simulink library "Common_Library"  (Simulink 8.1)
settings: Solver=ode45  StartTime=0.0  StopTime=10.0  RelTol=1e-3
values from neighbouring files (symbols this model uses):
  address_0x00 = MOVcr    [ROM.m]
  address_0x01 = 10    [ROM.m]
  address_0x02 = REG_A    [ROM.m]
  address_0x03 = MOVcr    [ROM.m]
  address_0x04 = 3    [ROM.m]
  address_0x05 = REG_B    [ROM.m]
  address_0x06 = ADDcr    [ROM.m]
  address_0x07 = 50    [ROM.m]
  address_0x08 = REG_B    [ROM.m]
  address_0x09 = ADDrr    [ROM.m]
  address_0x0A = REG_A    [ROM.m]
  address_0x0B = REG_B    [ROM.m]
  address_0x0C = 0    [ROM.m]
  address_0x0D = 0    [ROM.m]
  address_0x0E = 0    [ROM.m]
  address_0x0F = 177    [ROM.m]
libraries: Common_Library x115, Computer_Library x85, commutil2 x67, simulink_extras x1
(part 1 of 3)
settings Model: Creator=uzivatel  LastModifiedBy=uzivatel

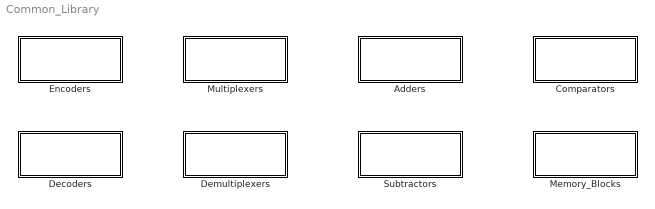
== system Common_Library ==
  Adders : Subsystem
  Comparators : Subsystem
  Decoders : Subsystem
  Demultiplexers : Subsystem
  Encoders : Subsystem
  Memory_Blocks : Subsystem
  Multiplexers : Subsystem
  Subtractors : Subsystem

== system Common_Library/Adders ==
  1_Bit_Adder : Subsystem
  1_Byte_Adder : Subsystem

== system Common_Library/Comparators ==
  1_Bit_Comparator : Subsystem
  1_Byte_Comparator : Subsystem

== system Common_Library/Decoders ==
  2_to_4_Decoder : Subsystem  TreatAsAtomicUnit=on
  3_to_8_Decoder : Subsystem  TreatAsAtomicUnit=on
  4_to_16_Decoder : Subsystem  RequirementInfo={} %GIDa_0eac4206_ee83_4851_a053_5bf277ce373a  TreatAsAtomicUnit=on
  __8_to_256_Decoder__ : Subsystem  Commented=on

== system Common_Library/Demultiplexers ==
  1_to_2_Bit_Demultiplexer : Subsystem
  1_to_2_Byte_Demultiplexer : Subsystem
  1_to_4_Bit_Demultiplexer : Subsystem
  1_to_4_Byte_Demultiplexer : Subsystem
  1_to_8_Bit_Demultiplexer : Subsystem
  1_to_8_Byte_Demultiplexer : Subsystem
  __1_to_16_Bit_Demultiplexer__ : Subsystem  Commented=on
  __1_to_16_Byte_Demultiplexer__ : Subsystem  Commented=on
  __1_to_256_Bit_Demultiplexer__ : Subsystem  Commented=on
  __1_to_256_Byte_Demultiplexer__ : Subsystem  Commented=on

== system Common_Library/Encoders ==
  4_to_2_Encoder : Subsystem
  __16_to_4_Encoder__ : Subsystem  Commented=on
  __8_to_3_Encoder__ : Subsystem  Commented=on

== system Common_Library/Memory_Blocks ==
  16B_RAM_Memory : Subsystem
  16B_ROM_Memory : Subsystem
  Bit : Subsystem
  Byte : Subsystem

== system Common_Library/Multiplexers ==
  16_to_1_Bit_Multiplexer : Subsystem
  16_to_1_Byte_Multiplexer : Subsystem
  2_to_1_Bit_Multiplexer : Subsystem
  2_to_1_Byte_Multiplexer : Subsystem
  4_to_1_Bit_Multiplexer : Subsystem
  4_to_1_Byte_Multiplexer : Subsystem
  8_to_1_Bit_Multiplexer : Subsystem
  8_to_1_Byte_Multiplexer : Subsystem
  __256_to_1_Bit_Multiplexer__ : Subsystem  Commented=on
  __256_to_1_Byte_Multiplexer__ : Subsystem  Commented=on

== system Common_Library/Subtractors ==
  1_Bit_Subtractor : Subsystem
  1_Byte_Subtractor : Subsystem

== system Common_Library/Adders/1_Bit_Adder ==
  Data_In_A(1b) : Inport
  Data_In_B(1b) : Inport  Port=2
  Carry_In(1b) : Inport  Port=3
  Logical Operator : Logic  IconShape=distinctive  AllPortsSameDT=off  OutDataTypeStr=boolean
  Logical Operator1 : Logic  IconShape=distinctive  AllPortsSameDT=off  OutDataTypeStr=boolean
  Logical Operator10 : Logic  Operator=NOT  Inputs=4  IconShape=distinctive  AllPortsSameDT=off  OutDataTypeStr=boolean
  Logical Operator11 : Logic  Operator=NOT  Inputs=4  IconShape=distinctive  AllPortsSameDT=off  OutDataTypeStr=boolean
  Logical Operator2 : Logic  IconShape=distinctive  AllPortsSameDT=off  OutDataTypeStr=boolean
  Logical Operator{3..6} (4 alike) : Logic  Inputs=3  IconShape=distinctive  AllPortsSameDT=off  OutDataTypeStr=boolean
  Logical Operator7 : Logic  Operator=OR  Inputs=4  IconShape=distinctive  AllPortsSameDT=off  OutDataTypeStr=boolean
  Logical Operator8 : Logic  Operator=OR  Inputs=3  IconShape=distinctive  AllPortsSameDT=off  OutDataTypeStr=boolean
  Logical Operator9 : Logic  Operator=NOT  Inputs=4  IconShape=distinctive  AllPortsSameDT=off  OutDataTypeStr=boolean
  Data_Out(1b) : Outport
  Carry_Out(1b) : Outport  Port=2
  wires:
  Logical Operator11/1 -> Logical Operator4/3, Logical Operator5/3
  Logical Operator10/1 -> Logical Operator3/2, Logical Operator5/2
  Logical Operator9/1 -> Logical Operator3/1, Logical Operator4/1
  Data_In_A(1b)/1 -> Logical Operator9/1, Logical Operator5/1, Logical Operator6/1, Logical Operator/1, Logical Operator1/1
  Data_In_B(1b)/1 -> Logical Operator10/1, Logical Operator4/2, Logical Operator6/2, Logical Operator/2, Logical Operator2/1
  Carry_In(1b)/1 -> Logical Operator11/1, Logical Operator3/3, Logical Operator6/3, Logical Operator1/2, Logical Operator2/2
  Logical Operator2/1 -> Logical Operator8/3
  Logical Operator1/1 -> Logical Operator8/2
  Logical Operator/1 -> Logical Operator8/1
  Logical Operator8/1 -> Carry_Out(1b)/1
  Logical Operator7/1 -> Data_Out(1b)/1
  Logical Operator6/1 -> Logical Operator7/4
  Logical Operator5/1 -> Logical Operator7/3
  Logical Operator4/1 -> Logical Operator7/2
  Logical Operator3/1 -> Logical Operator7/1

== system Common_Library/Adders/1_Byte_Adder ==
  Data_In_A(1B) : Inport
  Data_In_B(1B) : Inport  Port=2
  1_Bit_Adder{0..7} (8 alike) : Common_Library/Adders/1_Bit_Adder
  Bit to Integer Converter : commutil2/Bit to Integer Converter  nbits=8  bitOrder=MSB first  signedOutputValues=Unsigned  outDtype=uint8  outDtypeSigned=Inherit via internal rule
  Constant : Constant  Value=0
  Demux : Demux  Outputs=8
  Demux1 : Demux  Outputs=8
  Integer to Bit Converter : commutil2/Integer to Bit Converter  nbits=8  signedInputValues=Unsigned  bitOrder=MSB first  outDtype=uint8
  Integer to Bit Converter1 : commutil2/Integer to Bit Converter  nbits=8  signedInputValues=Unsigned  bitOrder=MSB first  outDtype=uint8
  Mux : Mux  Inputs=8
  Data_Out(1B) : Outport
  Carry_Out(1b) : Outport  Port=2
  wires:
  Bit to Integer Converter/1 -> Data_Out(1B)/1
  Mux/1 -> Bit to Integer Converter/1
  Integer to Bit Converter1/1 -> Demux1/1
  Data_In_B(1B)/1 -> Integer to Bit Converter1/1
  Integer to Bit Converter/1 -> Demux/1
  Data_In_A(1B)/1 -> Integer to Bit Converter/1
  1_Bit_Adder6/2 -> 1_Bit_Adder7/3
  1_Bit_Adder5/2 -> 1_Bit_Adder6/3
  1_Bit_Adder4/2 -> 1_Bit_Adder5/3
  1_Bit_Adder3/2 -> 1_Bit_Adder4/3
  1_Bit_Adder2/2 -> 1_Bit_Adder3/3
  1_Bit_Adder1/2 -> 1_Bit_Adder2/3
  1_Bit_Adder0/2 -> 1_Bit_Adder1/3
  1_Bit_Adder7/2 -> Carry_Out(1b)/1
  Constant/1 -> 1_Bit_Adder0/3
  Demux1/8 -> 1_Bit_Adder0/2
  Demux1/7 -> 1_Bit_Adder1/2
  Demux1/6 -> 1_Bit_Adder2/2
  Demux1/5 -> 1_Bit_Adder3/2
  Demux1/4 -> 1_Bit_Adder4/2
  Demux1/3 -> 1_Bit_Adder5/2
  Demux1/2 -> 1_Bit_Adder6/2
  Demux1/1 -> 1_Bit_Adder7/2
  Demux/8 -> 1_Bit_Adder0/1
  Demux/7 -> 1_Bit_Adder1/1
  Demux/6 -> 1_Bit_Adder2/1
  Demux/5 -> 1_Bit_Adder3/1
  Demux/4 -> 1_Bit_Adder4/1
  Demux/3 -> 1_Bit_Adder5/1
  Demux/2 -> 1_Bit_Adder6/1
  Demux/1 -> 1_Bit_Adder7/1
  1_Bit_Adder3/1 -> Mux/5
  1_Bit_Adder4/1 -> Mux/4
  1_Bit_Adder5/1 -> Mux/3
  1_Bit_Adder2/1 -> Mux/6
  1_Bit_Adder1/1 -> Mux/7
  1_Bit_Adder0/1 -> Mux/8
  1_Bit_Adder6/1 -> Mux/2
  1_Bit_Adder7/1 -> Mux/1

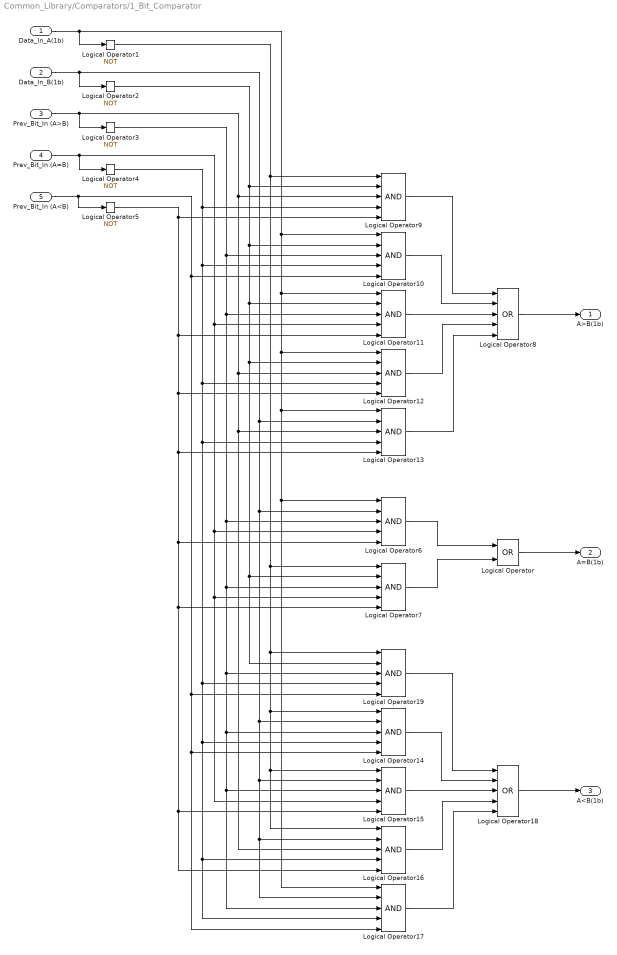
== system Common_Library/Comparators/1_Bit_Comparator ==
  Data_In_A(1b) : Inport
  Data_In_B(1b) : Inport  Port=2
  Prev_Bit_In (A>B) : Inport  Port=3
  Prev_Bit_In (A=B) : Inport  Port=4
  Prev_Bit_In (A<B) : Inport  Port=5
  Logical Operator : Logic  Operator=OR  IconShape=distinctive  AllPortsSameDT=off  OutDataTypeStr=boolean
  Logical Operator{1..5} (5 alike) : Logic  Operator=NOT  IconShape=distinctive  AllPortsSameDT=off  OutDataTypeStr=boolean
  Logical Operator{6..7,9..17,19} (12 alike) : Logic  Inputs=5  IconShape=distinctive  AllPortsSameDT=off  OutDataTypeStr=boolean
  Logical Operator18 : Logic  Operator=OR  Inputs=5  IconShape=distinctive  AllPortsSameDT=off  OutDataTypeStr=boolean
  Logical Operator8 : Logic  Operator=OR  Inputs=5  IconShape=distinctive  AllPortsSameDT=off  OutDataTypeStr=boolean
  A>B(1b) : Outport
  A=B(1b) : Outport  Port=2
  A<B(1b) : Outport  Port=3
  wires:
  Logical Operator16/1 -> Logical Operator18/4
  Logical Operator17/1 -> Logical Operator18/5
  Logical Operator19/1 -> Logical Operator18/1
  Logical Operator15/1 -> Logical Operator18/3
  Logical Operator14/1 -> Logical Operator18/2
  Logical Operator4/1 -> Logical Operator9/4, Logical Operator10/4, Logical Operator12/4, Logical Operator13/4, Logical Operator19/4, Logical Operator14/4, Logical Operator17/4, Logical Operator16/4
  Data_In_A(1b)/1 -> Logical Operator10/1, Logical Operator11/1, Logical Operator12/1, Logical Operator13/1, Logical Operator6/1, Logical Operator17/1, Logical Operator1/1
  Logical Operator5/1 -> Logical Operator9/5, Logical Operator11/5, Logical Operator12/5, Logical Operator13/5, Logical Operator6/5, Logical Operator7/5, Logical Operator15/5, Logical Operator16/5
  Logical Operator18/1 -> A<B(1b)/1
  Logical Operator2/1 -> Logical Operator9/2, Logical Operator10/2, Logical Operator11/2, Logical Operator12/2, Logical Operator7/2, Logical Operator19/2
  Logical Operator1/1 -> Logical Operator9/1, Logical Operator7/1, Logical Operator19/1, Logical Operator14/1, Logical Operator15/1, Logical Operator16/1
  Logical Operator3/1 -> Logical Operator10/3, Logical Operator11/3, Logical Operator6/3, Logical Operator7/3, Logical Operator19/3, Logical Operator14/3, Logical Operator15/3, Logical Operator17/3
  Prev_Bit_In (A<B)/1 -> Logical Operator5/1, Logical Operator10/5, Logical Operator19/5, Logical Operator14/5, Logical Operator17/5
  Prev_Bit_In (A>B)/1 -> Logical Operator3/1, Logical Operator9/3, Logical Operator12/3, Logical Operator13/3, Logical Operator16/3
  Prev_Bit_In (A=B)/1 -> Logical Operator11/4, Logical Operator6/4, Logical Operator7/4, Logical Operator15/4, Logical Operator4/1
  Logical Operator6/1 -> Logical Operator/1
  Logical Operator7/1 -> Logical Operator/2
  Data_In_B(1b)/1 -> Logical Operator2/1, Logical Operator13/2, Logical Operator6/2, Logical Operator17/2, Logical Operator16/2, Logical Operator15/2, Logical Operator14/2
  Logical Operator/1 -> A=B(1b)/1
  Logical Operator8/1 -> A>B(1b)/1
  Logical Operator13/1 -> Logical Operator8/5
  Logical Operator11/1 -> Logical Operator8/3
  Logical Operator10/1 -> Logical Operator8/2
  Logical Operator12/1 -> Logical Operator8/4
  Logical Operator9/1 -> Logical Operator8/1

== system Common_Library/Comparators/1_Byte_Comparator ==
  Data_In_A(1B) : Inport
  Data_In_B(1B) : Inport  Port=2
  1_Bit_Comparator{1..8} (8 alike) : Common_Library/Comparators/1_Bit_Comparator
  Constant3 : Constant  Value=0  OutDataTypeStr=int16
  Constant4 : Constant  OutDataTypeStr=int16
  Constant5 : Constant  Value=0  OutDataTypeStr=int16
  Demux1 : Demux  Outputs=8
  Demux2 : Demux  Outputs=8
  Integer to Bit Converter1 : commutil2/Integer to Bit Converter  nbits=8  signedInputValues=Unsigned  bitOrder=MSB first  outDtype=uint8
  Integer to Bit Converter2 : commutil2/Integer to Bit Converter  nbits=8  signedInputValues=Unsigned  bitOrder=MSB first  outDtype=uint8
  Saturation1 : Saturate  UpperLimit=255  LowerLimit=0
  Saturation2 : Saturate  UpperLimit=255  LowerLimit=0
  A>B(1b) : Outport
  A=B(1b) : Outport  Port=2
  A<B(1b) : Outport  Port=3
  wires:
  1_Bit_Comparator8/3 -> A<B(1b)/1
  1_Bit_Comparator8/1 -> A>B(1b)/1
  1_Bit_Comparator8/2 -> A=B(1b)/1
  Demux1/1 -> 1_Bit_Comparator8/1
  Demux1/2 -> 1_Bit_Comparator7/1
  Demux1/3 -> 1_Bit_Comparator6/1
  Demux1/4 -> 1_Bit_Comparator5/1
  Demux1/5 -> 1_Bit_Comparator4/1
  Demux1/6 -> 1_Bit_Comparator3/1
  Demux1/7 -> 1_Bit_Comparator2/1
  Data_In_A(1B)/1 -> Saturation1/1
  Saturation1/1 -> Integer to Bit Converter1/1
  Integer to Bit Converter1/1 -> Demux1/1
  Demux2/1 -> 1_Bit_Comparator8/2
  Demux2/2 -> 1_Bit_Comparator7/2
  Demux2/3 -> 1_Bit_Comparator6/2
  Demux2/4 -> 1_Bit_Comparator5/2
  Demux2/5 -> 1_Bit_Comparator4/2
  Demux2/6 -> 1_Bit_Comparator3/2
  Demux2/7 -> 1_Bit_Comparator2/2
  Data_In_B(1B)/1 -> Saturation2/1
  Saturation2/1 -> Integer to Bit Converter2/1
  Integer to Bit Converter2/1 -> Demux2/1
  1_Bit_Comparator7/3 -> 1_Bit_Comparator8/5
  1_Bit_Comparator7/2 -> 1_Bit_Comparator8/4
  1_Bit_Comparator7/1 -> 1_Bit_Comparator8/3
  1_Bit_Comparator6/3 -> 1_Bit_Comparator7/5
  1_Bit_Comparator6/2 -> 1_Bit_Comparator7/4
  1_Bit_Comparator6/1 -> 1_Bit_Comparator7/3
  1_Bit_Comparator5/3 -> 1_Bit_Comparator6/5
  1_Bit_Comparator5/2 -> 1_Bit_Comparator6/4
  1_Bit_Comparator5/1 -> 1_Bit_Comparator6/3
  1_Bit_Comparator4/3 -> 1_Bit_Comparator5/5
  1_Bit_Comparator4/2 -> 1_Bit_Comparator5/4
  1_Bit_Comparator4/1 -> 1_Bit_Comparator5/3
  1_Bit_Comparator3/3 -> 1_Bit_Comparator4/5
  1_Bit_Comparator3/2 -> 1_Bit_Comparator4/4
  1_Bit_Comparator3/1 -> 1_Bit_Comparator4/3
  1_Bit_Comparator2/3 -> 1_Bit_Comparator3/5
  1_Bit_Comparator2/1 -> 1_Bit_Comparator3/3
  1_Bit_Comparator2/2 -> 1_Bit_Comparator3/4
  Demux1/8 -> 1_Bit_Comparator1/1
  1_Bit_Comparator1/3 -> 1_Bit_Comparator2/5
  Demux2/8 -> 1_Bit_Comparator1/2
  Constant3/1 -> 1_Bit_Comparator1/3
  1_Bit_Comparator1/1 -> 1_Bit_Comparator2/3
  1_Bit_Comparator1/2 -> 1_Bit_Comparator2/4
  Constant5/1 -> 1_Bit_Comparator1/5
  Constant4/1 -> 1_Bit_Comparator1/4

== system Common_Library/Decoders/2_to_4_Decoder ==
  Address_1(1b) : Inport
  Address_0(1b) : Inport  Port=2
  Logical Operator{14..17} (4 alike) : Logic  IconShape=distinctive  AllPortsSameDT=off  OutDataTypeStr=boolean
  Logical Operator22 : Logic  Operator=NOT  IconShape=distinctive  AllPortsSameDT=off  OutDataTypeStr=boolean
  Logical Operator23 : Logic  Operator=NOT  IconShape=distinctive  AllPortsSameDT=off  OutDataTypeStr=boolean
  Select_3(1b) : Outport
  Select_2(1b) : Outport  Port=2
  Select_1(1b) : Outport  Port=3
  Select_0(1b) : Outport  Port=4
  wires:
  Address_0(1b)/1 -> Logical Operator23/1, Logical Operator16/2, Logical Operator14/1
  Logical Operator22/1 -> Logical Operator16/1, Logical Operator17/1
  Logical Operator23/1 -> Logical Operator15/1, Logical Operator17/2
  Address_1(1b)/1 -> Logical Operator14/2, Logical Operator15/2, Logical Operator22/1
  Logical Operator17/1 -> Select_0(1b)/1
  Logical Operator16/1 -> Select_1(1b)/1
  Logical Operator15/1 -> Select_2(1b)/1
  Logical Operator14/1 -> Select_3(1b)/1

== system Common_Library/Decoders/3_to_8_Decoder ==
  "Address_2(1b) " : Inport
  Address_1(1b) : Inport  Port=2
  Address_0(1b) : Inport  Port=3
  Logical Operator{10..17} (8 alike) : Logic  Inputs=3  IconShape=distinctive  AllPortsSameDT=off  OutDataTypeStr=boolean
  Logical Operator22 : Logic  Operator=NOT  IconShape=distinctive  AllPortsSameDT=off  OutDataTypeStr=boolean
  Logical Operator23 : Logic  Operator=NOT  IconShape=distinctive  AllPortsSameDT=off  OutDataTypeStr=boolean
  Logical Operator5 : Logic  Operator=NOT  IconShape=distinctive  AllPortsSameDT=off  OutDataTypeStr=boolean
  Select_7(1b) : Outport
  Select_6(1b) : Outport  Port=2
  Select_5(1b) : Outport  Port=3
  Select_4(1b) : Outport  Port=4
  Select_3(1b) : Outport  Port=5
  Select_2(1b) : Outport  Port=6
  Select_1(1b) : Outport  Port=7
  Select_0(1b) : Outport  Port=8
  wires:
  Address_0(1b)/1 -> Logical Operator10/3, Logical Operator12/3, Logical Operator14/3, Logical Operator16/2, Logical Operator23/1
  Logical Operator22/1 -> Logical Operator12/2, Logical Operator13/2, Logical Operator16/3, Logical Operator17/3
  Logical Operator23/1 -> Logical Operator11/3, Logical Operator13/3, Logical Operator15/3, Logical Operator17/2
  Logical Operator5/1 -> Logical Operator14/1, Logical Operator15/1, Logical Operator16/1, Logical Operator17/1
  Address_1(1b)/1 -> Logical Operator10/2, Logical Operator11/2, Logical Operator14/2, Logical Operator15/2, Logical Operator22/1
  "Address_2(1b) "/1 -> Logical Operator10/1, Logical Operator11/1, Logical Operator12/1, Logical Operator13/1, Logical Operator5/1
  Logical Operator17/1 -> Select_0(1b)/1
  Logical Operator16/1 -> Select_1(1b)/1
  Logical Operator15/1 -> Select_2(1b)/1
  Logical Operator14/1 -> Select_3(1b)/1
  Logical Operator13/1 -> Select_4(1b)/1
  Logical Operator12/1 -> Select_5(1b)/1
  Logical Operator11/1 -> Select_6(1b)/1
  Logical Operator10/1 -> Select_7(1b)/1

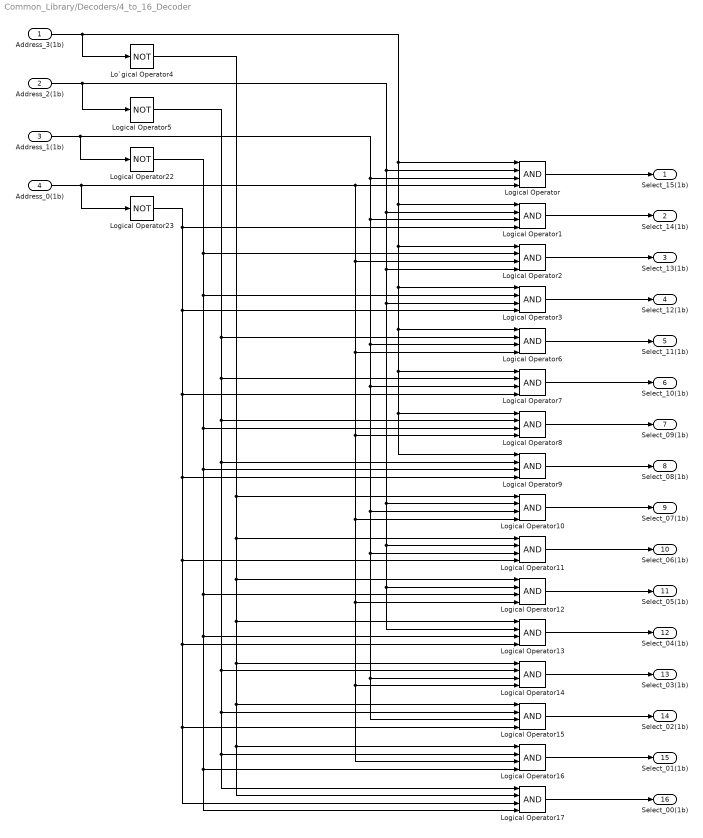
== system Common_Library/Decoders/4_to_16_Decoder ==
  Address_3(1b) : Inport
  "Address_2(1b) " : Inport  Port=2
  Address_1(1b) : Inport  Port=3
  Address_0(1b) : Inport  Port=4
  Lo`gical Operator4 : Logic  Operator=NOT  IconShape=distinctive  AllPortsSameDT=off  OutDataTypeStr=boolean
  Logical Operator{,1..3,6..17} (16 alike) : Logic  Inputs=4  IconShape=distinctive  AllPortsSameDT=off  OutDataTypeStr=boolean
  Logical Operator22 : Logic  Operator=NOT  IconShape=distinctive  AllPortsSameDT=off  OutDataTypeStr=boolean
  Logical Operator23 : Logic  Operator=NOT  IconShape=distinctive  AllPortsSameDT=off  OutDataTypeStr=boolean
  Logical Operator5 : Logic  Operator=NOT  IconShape=distinctive  AllPortsSameDT=off  OutDataTypeStr=boolean
  Select_15(1b) : Outport
  Select_14(1b) : Outport  Port=2
  Select_13(1b) : Outport  Port=3
  Select_12(1b) : Outport  Port=4
  Select_11(1b) : Outport  Port=5
  Select_10(1b) : Outport  Port=6
  Select_09(1b) : Outport  Port=7
  Select_08(1b) : Outport  Port=8
  Select_07(1b) : Outport  Port=9
  Select_06(1b) : Outport  Port=10
  Select_05(1b) : Outport  Port=11
  Select_04(1b) : Outport  Port=12
  Select_03(1b) : Outport  Port=13
  Select_02(1b) : Outport  Port=14
  Select_01(1b) : Outport  Port=15
  Select_00(1b) : Outport  Port=16
  wires:
  Logical Operator22/1 -> Logical Operator2/2, Logical Operator3/2, Logical Operator8/3, Logical Operator9/3, Logical Operator12/3, Logical Operator13/3, Logical Operator16/4, Logical Operator17/4
  Address_0(1b)/1 -> Logical Operator/4, Logical Operator2/3, Logical Operator6/4, Logical Operator8/4, Logical Operator10/4, Logical Operator12/4, Logical Operator14/4, Logical Operator16/3, Logical Operator23/1
  Logical Operator23/1 -> Logical Operator1/4, Logical Operator3/4, Logical Operator7/4, Logical Operator9/4, Logical Operator11/4, Logical Operator13/4, Logical Operator15/4, Logical Operator17/3
  Logical Operator5/1 -> Logical Operator6/2, Logical Operator7/2, Logical Operator8/2, Logical Operator9/2, Logical Operator14/2, Logical Operator15/2, Logical Operator16/2, Logical Operator17/1
  Address_3(1b)/1 -> Lo`gical Operator4/1, Logical Operator2/1, Logical Operator3/1, Logical Operator6/1, Logical Operator7/1, Logical Operator8/1, Logical Operator9/1, Logical Operator1/1, Logical Operator/1
  Address_1(1b)/1 -> Logical Operator22/1, Logical Operator/3, Logical Operator1/3, Logical Operator6/3, Logical Operator7/3, Logical Operator10/3, Logical Operator11/3, Logical Operator14/3, Logical Operator15/3
  "Address_2(1b) "/1 -> Logical Operator/2, Logical Operator1/2, Logical Operator2/4, Logical Operator3/3, Logical Operator10/2, Logical Operator11/2, Logical Operator12/2, Logical Operator13/2, Logical Operator5/1
  Lo`gical Operator4/1 -> Logical Operator10/1, Logical Operator11/1, Logical Operator12/1, Logical Operator13/1, Logical Operator14/1, Logical Operator15/1, Logical Operator16/1, Logical Operator17/2
  Logical Operator17/1 -> Select_00(1b)/1
  Logical Operator16/1 -> Select_01(1b)/1
  Logical Operator15/1 -> Select_02(1b)/1
  Logical Operator14/1 -> Select_03(1b)/1
  Logical Operator13/1 -> Select_04(1b)/1
  Logical Operator12/1 -> Select_05(1b)/1
  Logical Operator11/1 -> Select_06(1b)/1
  Logical Operator10/1 -> Select_07(1b)/1
  Logical Operator9/1 -> Select_08(1b)/1
  Logical Operator8/1 -> Select_09(1b)/1
  Logical Operator7/1 -> Select_10(1b)/1
  Logical Operator6/1 -> Select_11(1b)/1
  Logical Operator1/1 -> Select_14(1b)/1
  Logical Operator2/1 -> Select_13(1b)/1
  Logical Operator3/1 -> Select_12(1b)/1
  Logical Operator/1 -> Select_15(1b)/1

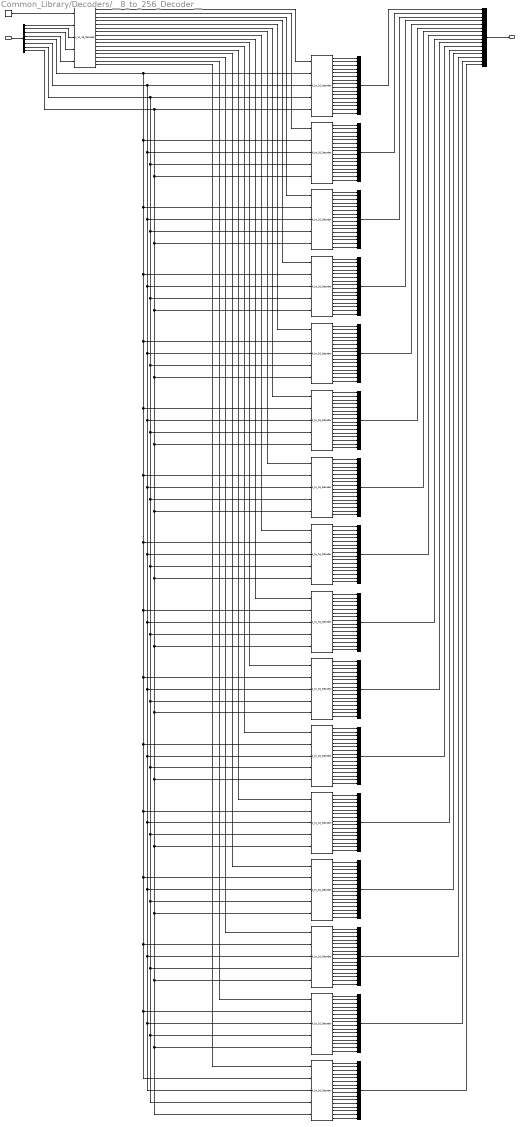
== system Common_Library/Decoders/__8_to_256_Decoder__ ==
  Address(8b) : Inport
  4_to_16_Decoder{,1..16} (17 alike) : Computer_Library/4_to_16_Decoder
  Demux : Demux  Outputs=8
  Enable : Constant
  Mux{,1..16} (17 alike) : Mux  Inputs=16
  Select_Byte(256b) : Outport
  wires:
  Mux/1 -> Select_Byte(256b)/1
  Address(8b)/1 -> Demux/1
  Mux2/1 -> Mux/2
  Mux3/1 -> Mux/3
  Mux4/1 -> Mux/4
  Mux5/1 -> Mux/5
  Mux6/1 -> Mux/6
  Mux7/1 -> Mux/7
  Mux8/1 -> Mux/8
  Mux9/1 -> Mux/9
  Mux10/1 -> Mux/10
  Mux11/1 -> Mux/11
  Mux12/1 -> Mux/12
  Mux13/1 -> Mux/13
  Mux14/1 -> Mux/14
  Mux15/1 -> Mux/15
  Mux16/1 -> Mux/16
  Mux1/1 -> Mux/1
  4_to_16_Decoder16/16 -> Mux16/16
  4_to_16_Decoder16/15 -> Mux16/15
  4_to_16_Decoder16/14 -> Mux16/14
  4_to_16_Decoder16/13 -> Mux16/13
  4_to_16_Decoder16/12 -> Mux16/12
  4_to_16_Decoder16/11 -> Mux16/11
  4_to_16_Decoder16/10 -> Mux16/10
  4_to_16_Decoder16/9 -> Mux16/9
  4_to_16_Decoder16/8 -> Mux16/8
  4_to_16_Decoder16/7 -> Mux16/7
  4_to_16_Decoder16/6 -> Mux16/6
  4_to_16_Decoder16/5 -> Mux16/5
  4_to_16_Decoder16/4 -> Mux16/4
  4_to_16_Decoder16/3 -> Mux16/3
  4_to_16_Decoder16/2 -> Mux16/2
  4_to_16_Decoder16/1 -> Mux16/1
  4_to_16_Decoder15/16 -> Mux15/16
  4_to_16_Decoder15/15 -> Mux15/15
  4_to_16_Decoder15/14 -> Mux15/14
  4_to_16_Decoder15/13 -> Mux15/13
  4_to_16_Decoder15/12 -> Mux15/12
  4_to_16_Decoder15/11 -> Mux15/11
  4_to_16_Decoder15/10 -> Mux15/10
  4_to_16_Decoder15/9 -> Mux15/9
  4_to_16_Decoder15/8 -> Mux15/8
  4_to_16_Decoder15/7 -> Mux15/7
  4_to_16_Decoder15/6 -> Mux15/6
  4_to_16_Decoder15/5 -> Mux15/5
  4_to_16_Decoder15/4 -> Mux15/4
  4_to_16_Decoder15/3 -> Mux15/3
  4_to_16_Decoder15/2 -> Mux15/2
  4_to_16_Decoder15/1 -> Mux15/1
  4_to_16_Decoder14/16 -> Mux14/16
  4_to_16_Decoder14/15 -> Mux14/15
  4_to_16_Decoder14/14 -> Mux14/14
  4_to_16_Decoder14/13 -> Mux14/13
  4_to_16_Decoder14/12 -> Mux14/12
  4_to_16_Decoder14/11 -> Mux14/11
  4_to_16_Decoder14/10 -> Mux14/10
  4_to_16_Decoder14/9 -> Mux14/9
  4_to_16_Decoder14/8 -> Mux14/8
  4_to_16_Decoder14/7 -> Mux14/7
  4_to_16_Decoder14/6 -> Mux14/6
  4_to_16_Decoder14/5 -> Mux14/5
  4_to_16_Decoder14/4 -> Mux14/4
  4_to_16_Decoder14/3 -> Mux14/3
  4_to_16_Decoder14/2 -> Mux14/2
  4_to_16_Decoder14/1 -> Mux14/1
  4_to_16_Decoder13/16 -> Mux13/16
  4_to_16_Decoder13/15 -> Mux13/15
  4_to_16_Decoder13/14 -> Mux13/14
  4_to_16_Decoder13/13 -> Mux13/13
  4_to_16_Decoder13/12 -> Mux13/12
  4_to_16_Decoder13/11 -> Mux13/11
  4_to_16_Decoder13/10 -> Mux13/10
  4_to_16_Decoder13/9 -> Mux13/9
  4_to_16_Decoder13/8 -> Mux13/8
  4_to_16_Decoder13/7 -> Mux13/7
  4_to_16_Decoder13/6 -> Mux13/6
  4_to_16_Decoder13/5 -> Mux13/5
  4_to_16_Decoder13/4 -> Mux13/4
  4_to_16_Decoder13/3 -> Mux13/3
  4_to_16_Decoder13/2 -> Mux13/2
  4_to_16_Decoder13/1 -> Mux13/1
  4_to_16_Decoder12/16 -> Mux12/16
  4_to_16_Decoder12/15 -> Mux12/15
  4_to_16_Decoder12/14 -> Mux12/14
  4_to_16_Decoder12/13 -> Mux12/13
  4_to_16_Decoder12/12 -> Mux12/12
  4_to_16_Decoder12/11 -> Mux12/11
  4_to_16_Decoder12/10 -> Mux12/10
  4_to_16_Decoder12/9 -> Mux12/9
  4_to_16_Decoder12/8 -> Mux12/8
  4_to_16_Decoder12/7 -> Mux12/7
  4_to_16_Decoder12/6 -> Mux12/6
  4_to_16_Decoder12/5 -> Mux12/5
  4_to_16_Decoder12/4 -> Mux12/4
  4_to_16_Decoder12/3 -> Mux12/3
  4_to_16_Decoder12/2 -> Mux12/2
  4_to_16_Decoder12/1 -> Mux12/1
  4_to_16_Decoder11/16 -> Mux11/16
  4_to_16_Decoder11/15 -> Mux11/15
  4_to_16_Decoder11/14 -> Mux11/14
  4_to_16_Decoder11/13 -> Mux11/13
  4_to_16_Decoder11/12 -> Mux11/12
  4_to_16_Decoder11/11 -> Mux11/11
  4_to_16_Decoder11/10 -> Mux11/10
  4_to_16_Decoder11/9 -> Mux11/9
  4_to_16_Decoder11/8 -> Mux11/8
  4_to_16_Decoder11/7 -> Mux11/7
  4_to_16_Decoder11/6 -> Mux11/6
  4_to_16_Decoder11/5 -> Mux11/5
  4_to_16_Decoder11/4 -> Mux11/4
  4_to_16_Decoder11/3 -> Mux11/3
  4_to_16_Decoder11/2 -> Mux11/2
  4_to_16_Decoder11/1 -> Mux11/1
  4_to_16_Decoder10/16 -> Mux10/16
  4_to_16_Decoder10/15 -> Mux10/15
  4_to_16_Decoder10/14 -> Mux10/14
  4_to_16_Decoder10/13 -> Mux10/13
  4_to_16_Decoder10/12 -> Mux10/12
  4_to_16_Decoder10/11 -> Mux10/11
  4_to_16_Decoder10/10 -> Mux10/10
  4_to_16_Decoder10/9 -> Mux10/9
  4_to_16_Decoder10/8 -> Mux10/8
  4_to_16_Decoder10/7 -> Mux10/7
  4_to_16_Decoder10/6 -> Mux10/6
  4_to_16_Decoder10/5 -> Mux10/5
  4_to_16_Decoder10/4 -> Mux10/4
  4_to_16_Decoder10/3 -> Mux10/3
  4_to_16_Decoder10/2 -> Mux10/2
  4_to_16_Decoder10/1 -> Mux10/1
  4_to_16_Decoder9/16 -> Mux9/16
  4_to_16_Decoder9/15 -> Mux9/15
  4_to_16_Decoder9/14 -> Mux9/14
  4_to_16_Decoder9/13 -> Mux9/13
  4_to_16_Decoder9/12 -> Mux9/12
  4_to_16_Decoder9/11 -> Mux9/11
  4_to_16_Decoder9/10 -> Mux9/10
  4_to_16_Decoder9/9 -> Mux9/9
  4_to_16_Decoder9/8 -> Mux9/8
  4_to_16_Decoder9/7 -> Mux9/7
  4_to_16_Decoder9/6 -> Mux9/6
  4_to_16_Decoder9/5 -> Mux9/5
  4_to_16_Decoder9/4 -> Mux9/4
  4_to_16_Decoder9/3 -> Mux9/3
  4_to_16_Decoder9/2 -> Mux9/2
  4_to_16_Decoder9/1 -> Mux9/1
  4_to_16_Decoder8/16 -> Mux8/16
  4_to_16_Decoder8/15 -> Mux8/15
  4_to_16_Decoder8/14 -> Mux8/14
  4_to_16_Decoder8/13 -> Mux8/13
  4_to_16_Decoder8/12 -> Mux8/12
  4_to_16_Decoder8/11 -> Mux8/11
  4_to_16_Decoder8/10 -> Mux8/10
  4_to_16_Decoder8/9 -> Mux8/9
  4_to_16_Decoder8/8 -> Mux8/8
  4_to_16_Decoder8/7 -> Mux8/7
  4_to_16_Decoder8/6 -> Mux8/6
  4_to_16_Decoder8/5 -> Mux8/5
  4_to_16_Decoder8/4 -> Mux8/4
  4_to_16_Decoder8/3 -> Mux8/3
  4_to_16_Decoder8/2 -> Mux8/2
  4_to_16_Decoder8/1 -> Mux8/1
  4_to_16_Decoder7/16 -> Mux7/16
  4_to_16_Decoder7/15 -> Mux7/15
  4_to_16_Decoder7/14 -> Mux7/14
  4_to_16_Decoder7/13 -> Mux7/13
  4_to_16_Decoder7/12 -> Mux7/12
  4_to_16_Decoder7/11 -> Mux7/11
  4_to_16_Decoder7/10 -> Mux7/10
  4_to_16_Decoder7/9 -> Mux7/9
  4_to_16_Decoder7/8 -> Mux7/8
  4_to_16_Decoder7/7 -> Mux7/7
  4_to_16_Decoder7/6 -> Mux7/6
  4_to_16_Decoder7/5 -> Mux7/5
  4_to_16_Decoder7/4 -> Mux7/4
  4_to_16_Decoder7/3 -> Mux7/3
  4_to_16_Decoder7/2 -> Mux7/2
  4_to_16_Decoder7/1 -> Mux7/1
  4_to_16_Decoder6/16 -> Mux6/16
  4_to_16_Decoder6/15 -> Mux6/15
  4_to_16_Decoder6/14 -> Mux6/14
  4_to_16_Decoder6/13 -> Mux6/13
  4_to_16_Decoder6/12 -> Mux6/12
  4_to_16_Decoder6/11 -> Mux6/11
  4_to_16_Decoder6/10 -> Mux6/10
  4_to_16_Decoder6/9 -> Mux6/9
  4_to_16_Decoder6/8 -> Mux6/8
  4_to_16_Decoder6/7 -> Mux6/7
  4_to_16_Decoder6/6 -> Mux6/6
  4_to_16_Decoder6/5 -> Mux6/5
  4_to_16_Decoder6/4 -> Mux6/4
  4_to_16_Decoder6/3 -> Mux6/3
  4_to_16_Decoder6/2 -> Mux6/2
  4_to_16_Decoder6/1 -> Mux6/1
  4_to_16_Decoder5/16 -> Mux5/16
  4_to_16_Decoder5/15 -> Mux5/15
  4_to_16_Decoder5/14 -> Mux5/14
  4_to_16_Decoder5/13 -> Mux5/13
  4_to_16_Decoder5/12 -> Mux5/12
  4_to_16_Decoder5/11 -> Mux5/11
  4_to_16_Decoder5/10 -> Mux5/10
  4_to_16_Decoder5/9 -> Mux5/9
  4_to_16_Decoder5/8 -> Mux5/8
  4_to_16_Decoder5/7 -> Mux5/7
  4_to_16_Decoder5/6 -> Mux5/6
  4_to_16_Decoder5/5 -> Mux5/5
  4_to_16_Decoder5/4 -> Mux5/4
  4_to_16_Decoder5/3 -> Mux5/3
  4_to_16_Decoder5/2 -> Mux5/2
  4_to_16_Decoder5/1 -> Mux5/1
  4_to_16_Decoder4/16 -> Mux4/16
  4_to_16_Decoder4/15 -> Mux4/15
  4_to_16_Decoder4/14 -> Mux4/14
  4_to_16_Decoder4/13 -> Mux4/13
  4_to_16_Decoder4/12 -> Mux4/12
  4_to_16_Decoder4/11 -> Mux4/11
  4_to_16_Decoder4/10 -> Mux4/10
  4_to_16_Decoder4/9 -> Mux4/9
  4_to_16_Decoder4/8 -> Mux4/8
  4_to_16_Decoder4/7 -> Mux4/7
  4_to_16_Decoder4/6 -> Mux4/6
  4_to_16_Decoder4/5 -> Mux4/5
  4_to_16_Decoder4/4 -> Mux4/4
  4_to_16_Decoder4/3 -> Mux4/3
  4_to_16_Decoder4/2 -> Mux4/2
  4_to_16_Decoder4/1 -> Mux4/1
  4_to_16_Decoder3/16 -> Mux3/16
  4_to_16_Decoder3/15 -> Mux3/15
  4_to_16_Decoder3/14 -> Mux3/14
  4_to_16_Decoder3/13 -> Mux3/13
  4_to_16_Decoder3/12 -> Mux3/12
  4_to_16_Decoder3/11 -> Mux3/11
  4_to_16_Decoder3/10 -> Mux3/10
  4_to_16_Decoder3/9 -> Mux3/9
  4_to_16_Decoder3/8 -> Mux3/8
  4_to_16_Decoder3/7 -> Mux3/7
  4_to_16_Decoder3/6 -> Mux3/6
  4_to_16_Decoder3/5 -> Mux3/5
  4_to_16_Decoder3/4 -> Mux3/4
  4_to_16_Decoder3/3 -> Mux3/3
  4_to_16_Decoder3/2 -> Mux3/2
  4_to_16_Decoder3/1 -> Mux3/1
  4_to_16_Decoder2/16 -> Mux2/16
  4_to_16_Decoder2/15 -> Mux2/15
  4_to_16_Decoder2/14 -> Mux2/14
  4_to_16_Decoder2/13 -> Mux2/13
  4_to_16_Decoder2/12 -> Mux2/12
  4_to_16_Decoder2/11 -> Mux2/11
  4_to_16_Decoder2/10 -> Mux2/10
  4_to_16_Decoder2/9 -> Mux2/9
  4_to_16_Decoder2/8 -> Mux2/8
  4_to_16_Decoder2/7 -> Mux2/7
  4_to_16_Decoder2/6 -> Mux2/6
  4_to_16_Decoder2/5 -> Mux2/5
  4_to_16_Decoder2/4 -> Mux2/4
  4_to_16_Decoder2/3 -> Mux2/3
  4_to_16_Decoder2/2 -> Mux2/2
  4_to_16_Decoder2/1 -> Mux2/1
  4_to_16_Decoder1/16 -> Mux1/16
  4_to_16_Decoder1/15 -> Mux1/15
  4_to_16_Decoder1/14 -> Mux1/14
  4_to_16_Decoder1/13 -> Mux1/13
  4_to_16_Decoder1/12 -> Mux1/12
  4_to_16_Decoder1/11 -> Mux1/11
  4_to_16_Decoder1/10 -> Mux1/10
  4_to_16_Decoder1/9 -> Mux1/9
  4_to_16_Decoder1/8 -> Mux1/8
  4_to_16_Decoder1/7 -> Mux1/7
  4_to_16_Decoder1/6 -> Mux1/6
  4_to_16_Decoder1/5 -> Mux1/5
  4_to_16_Decoder1/4 -> Mux1/4
  4_to_16_Decoder1/3 -> Mux1/3
  4_to_16_Decoder1/2 -> Mux1/2
  4_to_16_Decoder1/1 -> Mux1/1
  Enable/1 -> 4_to_16_Decoder/1
  4_to_16_Decoder/16 -> 4_to_16_Decoder16/1
  4_to_16_Decoder/15 -> 4_to_16_Decoder15/1
  4_to_16_Decoder/14 -> 4_to_16_Decoder14/1
  4_to_16_Decoder/13 -> 4_to_16_Decoder13/1
  4_to_16_Decoder/12 -> 4_to_16_Decoder12/1
  4_to_16_Decoder/11 -> 4_to_16_Decoder11/1
  4_to_16_Decoder/10 -> 4_to_16_Decoder10/1
  4_to_16_Decoder/9 -> 4_to_16_Decoder9/1
  4_to_16_Decoder/8 -> 4_to_16_Decoder8/1
  4_to_16_Decoder/7 -> 4_to_16_Decoder7/1
  4_to_16_Decoder/6 -> 4_to_16_Decoder6/1
  4_to_16_Decoder/5 -> 4_to_16_Decoder5/1
  4_to_16_Decoder/4 -> 4_to_16_Decoder4/1
  4_to_16_Decoder/3 -> 4_to_16_Decoder3/1
  4_to_16_Decoder/2 -> 4_to_16_Decoder2/1
  4_to_16_Decoder/1 -> 4_to_16_Decoder1/1
  Demux/8 -> 4_to_16_Decoder15/5, 4_to_16_Decoder16/5, 4_to_16_Decoder14/5, 4_to_16_Decoder13/5, 4_to_16_Decoder12/5, 4_to_16_Decoder11/5, 4_to_16_Decoder10/5, 4_to_16_Decoder9/5, 4_to_16_Decoder8/5, 4_to_16_Decoder7/5, 4_to_16_Decoder6/5, 4_to_16_Decoder5/5, 4_to_16_Decoder4/5, 4_to_16_Decoder3/5, 4_to_16_Decoder2/5, 4_to_16_Decoder1/5
  Demux/7 -> 4_to_16_Decoder15/4, 4_to_16_Decoder16/4, 4_to_16_Decoder14/4, 4_to_16_Decoder13/4, 4_to_16_Decoder12/4, 4_to_16_Decoder11/4, 4_to_16_Decoder10/4, 4_to_16_Decoder9/4, 4_to_16_Decoder8/4, 4_to_16_Decoder7/4, 4_to_16_Decoder6/4, 4_to_16_Decoder5/4, 4_to_16_Decoder4/4, 4_to_16_Decoder3/4, 4_to_16_Decoder2/4, 4_to_16_Decoder1/4
  Demux/6 -> 4_to_16_Decoder15/3, 4_to_16_Decoder16/3, 4_to_16_Decoder14/3, 4_to_16_Decoder13/3, 4_to_16_Decoder12/3, 4_to_16_Decoder11/3, 4_to_16_Decoder10/3, 4_to_16_Decoder9/3, 4_to_16_Decoder8/3, 4_to_16_Decoder7/3, 4_to_16_Decoder6/3, 4_to_16_Decoder5/3, 4_to_16_Decoder4/3, 4_to_16_Decoder3/3, 4_to_16_Decoder2/3, 4_to_16_Decoder1/3
  Demux/5 -> 4_to_16_Decoder15/2, 4_to_16_Decoder16/2, 4_to_16_Decoder14/2, 4_to_16_Decoder13/2, 4_to_16_Decoder12/2, 4_to_16_Decoder11/2, 4_to_16_Decoder10/2, 4_to_16_Decoder9/2, 4_to_16_Decoder8/2, 4_to_16_Decoder7/2, 4_to_16_Decoder6/2, 4_to_16_Decoder5/2, 4_to_16_Decoder4/2, 4_to_16_Decoder3/2, 4_to_16_Decoder2/2, 4_to_16_Decoder1/2
  Demux/4 -> 4_to_16_Decoder/5
  Demux/3 -> 4_to_16_Decoder/4
  Demux/2 -> 4_to_16_Decoder/3
  Demux/1 -> 4_to_16_Decoder/2

== system Common_Library/Demultiplexers/1_to_2_Bit_Demultiplexer ==
  Address(1b) : Inport
  Data_In(1b) : Inport  Port=2
  Logical Operator2 : Logic  IconShape=distinctive  AllPortsSameDT=off  OutDataTypeStr=boolean
  Logical Operator22 : Logic  Operator=NOT  Inputs=4  IconShape=distinctive  AllPortsSameDT=off  OutDataTypeStr=boolean
  Logical Operator3 : Logic  IconShape=distinctive  AllPortsSameDT=off  OutDataTypeStr=boolean
  Data_Out_1(1b) : Outport
  Data_Out_0(1b) : Outport  Port=2
  wires:
  Logical Operator3/1 -> Data_Out_0(1b)/1
  Logical Operator2/1 -> Data_Out_1(1b)/1
  Logical Operator22/1 -> Logical Operator3/2
  Address(1b)/1 -> Logical Operator2/2, Logical Operator22/1
  Data_In(1b)/1 -> Logical Operator2/1, Logical Operator3/1

== system Common_Library/Demultiplexers/1_to_2_Byte_Demultiplexer ==
  Address(1b) : Inport
  Data_In(1B) : Inport  Port=2
  1_to_2_Bit_Demultiplexer{,1..7} (8 alike) : Common_Library/Demultiplexers/1_to_2_Bit_Demultiplexer
  Bit to Integer Converter2 : commutil2/Bit to Integer Converter  nbits=8  bitOrder=MSB first  signedOutputValues=Unsigned  outDtype=uint8  outDtypeSigned=Inherit via internal rule
  Bit to Integer Converter3 : commutil2/Bit to Integer Converter  nbits=8  bitOrder=MSB first  signedOutputValues=Unsigned  outDtype=uint8  outDtypeSigned=Inherit via internal rule
  Byte_0 : Mux  Inputs=8
  Byte_1 : Mux  Inputs=8
  Demux1 : Demux  Outputs=8
  Integer to Bit Converter7 : commutil2/Integer to Bit Converter  nbits=8  signedInputValues=Unsigned  bitOrder=MSB first  outDtype=boolean
  Data_Out_1(1B) : Outport
  Data_Out_0(1B) : Outport  Port=2
  wires:
  Demux1/4 -> 1_to_2_Bit_Demultiplexer3/2
  Demux1/5 -> 1_to_2_Bit_Demultiplexer4/2
  Demux1/6 -> 1_to_2_Bit_Demultiplexer5/2
  Demux1/7 -> 1_to_2_Bit_Demultiplexer6/2
  Demux1/8 -> 1_to_2_Bit_Demultiplexer7/2
  Demux1/3 -> 1_to_2_Bit_Demultiplexer2/2
  Demux1/2 -> 1_to_2_Bit_Demultiplexer1/2
  Demux1/1 -> 1_to_2_Bit_Demultiplexer/2
  Byte_1/1 -> Bit to Integer Converter2/1
  Byte_0/1 -> Bit to Integer Converter3/1
  1_to_2_Bit_Demultiplexer7/2 -> Byte_0/8
  1_to_2_Bit_Demultiplexer7/1 -> Byte_1/8
  1_to_2_Bit_Demultiplexer6/2 -> Byte_0/7
  1_to_2_Bit_Demultiplexer6/1 -> Byte_1/7
  1_to_2_Bit_Demultiplexer5/2 -> Byte_0/6
  1_to_2_Bit_Demultiplexer5/1 -> Byte_1/6
  1_to_2_Bit_Demultiplexer4/2 -> Byte_0/5
  1_to_2_Bit_Demultiplexer4/1 -> Byte_1/5
  1_to_2_Bit_Demultiplexer3/2 -> Byte_0/4
  1_to_2_Bit_Demultiplexer3/1 -> Byte_1/4
  1_to_2_Bit_Demultiplexer2/2 -> Byte_0/3
  1_to_2_Bit_Demultiplexer2/1 -> Byte_1/3
  1_to_2_Bit_Demultiplexer1/2 -> Byte_0/2
  1_to_2_Bit_Demultiplexer1/1 -> Byte_1/2
  1_to_2_Bit_Demultiplexer/2 -> Byte_0/1
  1_to_2_Bit_Demultiplexer/1 -> Byte_1/1
  Integer to Bit Converter7/1 -> Demux1/1
  Data_In(1B)/1 -> Integer to Bit Converter7/1
  Address(1b)/1 -> 1_to_2_Bit_Demultiplexer/1, 1_to_2_Bit_Demultiplexer7/1, 1_to_2_Bit_Demultiplexer6/1, 1_to_2_Bit_Demultiplexer5/1, 1_to_2_Bit_Demultiplexer4/1, 1_to_2_Bit_Demultiplexer3/1, 1_to_2_Bit_Demultiplexer2/1, 1_to_2_Bit_Demultiplexer1/1
  Bit to Integer Converter2/1 -> Data_Out_1(1B)/1
  Bit to Integer Converter3/1 -> Data_Out_0(1B)/1

== system Common_Library/Demultiplexers/1_to_4_Bit_Demultiplexer ==
  Address_1(1b) : Inport
  Address_0(1b) : Inport  Port=2
  Data_In(1b) : Inport  Port=3
  Logical Operator{,1..3} (4 alike) : Logic  Inputs=3  IconShape=distinctive  AllPortsSameDT=off  OutDataTypeStr=boolean
  Logical Operator21 : Logic  Operator=NOT  Inputs=4  IconShape=distinctive  AllPortsSameDT=off  OutDataTypeStr=boolean
  Logical Operator22 : Logic  Operator=NOT  Inputs=4  IconShape=distinctive  AllPortsSameDT=off  OutDataTypeStr=boolean
  Data_Out_3(1b) : Outport
  Data_Out_2(1b) : Outport  Port=2
  Data_Out_1(1b) : Outport  Port=3
  Data_Out_0(1b) : Outport  Port=4
  wires:
  Logical Operator3/1 -> Data_Out_0(1b)/1
  Logical Operator2/1 -> Data_Out_1(1b)/1
  Logical Operator1/1 -> Data_Out_2(1b)/1
  Logical Operator/1 -> Data_Out_3(1b)/1
  Logical Operator22/1 -> Logical Operator1/2, Logical Operator3/2
  Address_0(1b)/1 -> Logical Operator2/2, Logical Operator/2, Logical Operator22/1
  Logical Operator21/1 -> Logical Operator2/3, Logical Operator3/3
  Address_1(1b)/1 -> Logical Operator1/3, Logical Operator/3, Logical Operator21/1
  Data_In(1b)/1 -> Logical Operator/1, Logical Operator1/1, Logical Operator2/1, Logical Operator3/1

== system Common_Library/Demultiplexers/1_to_4_Byte_Demultiplexer ==
  Address_1(1b) : Inport
  Address_0(1b) : Inport  Port=2
  Data_In(1B) : Inport  Port=3
  1_to_4_Bit_Demultiplexer(Bit_0) : Common_Library/Demultiplexers/1_to_4_Bit_Demultiplexer
  1_to_4_Bit_Demultiplexer(Bit_1) : Common_Library/Demultiplexers/1_to_4_Bit_Demultiplexer
  1_to_4_Bit_Demultiplexer(Bit_2) : Common_Library/Demultiplexers/1_to_4_Bit_Demultiplexer
  1_to_4_Bit_Demultiplexer(Bit_3) : Common_Library/Demultiplexers/1_to_4_Bit_Demultiplexer
  1_to_4_Bit_Demultiplexer(Bit_4) : Common_Library/Demultiplexers/1_to_4_Bit_Demultiplexer
  1_to_4_Bit_Demultiplexer(Bit_5) : Common_Library/Demultiplexers/1_to_4_Bit_Demultiplexer
  1_to_4_Bit_Demultiplexer(Bit_6) : Common_Library/Demultiplexers/1_to_4_Bit_Demultiplexer
  1_to_4_Bit_Demultiplexer(Bit_7) : Common_Library/Demultiplexers/1_to_4_Bit_Demultiplexer
  Bit to Integer Converter{,1..3} (4 alike) : commutil2/Bit to Integer Converter  nbits=8  bitOrder=MSB first  signedOutputValues=Unsigned  outDtype=uint8  outDtypeSigned=Inherit via internal rule
  Byte_{0..3} (4 alike) : Mux  Inputs=8
  Demux1 : Demux  Outputs=8
  Integer to Bit Converter7 : commutil2/Integer to Bit Converter  nbits=8  signedInputValues=Unsigned  bitOrder=MSB first  outDtype=boolean
  Data_Out_3(1B) : Outport
  Data_Out_2(1B) : Outport  Port=2
  Data_Out_1(1B) : Outport  Port=3
  Data_Out_0(1B) : Outport  Port=4
  wires:
  Bit to Integer Converter/1 -> Data_Out_3(1B)/1
  Demux1/4 -> 1_to_4_Bit_Demultiplexer(Bit_4)/3
  Demux1/5 -> 1_to_4_Bit_Demultiplexer(Bit_3)/3
  Demux1/6 -> 1_to_4_Bit_Demultiplexer(Bit_2)/3
  Demux1/7 -> 1_to_4_Bit_Demultiplexer(Bit_1)/3
  Demux1/8 -> 1_to_4_Bit_Demultiplexer(Bit_0)/3
  Demux1/3 -> 1_to_4_Bit_Demultiplexer(Bit_5)/3
  Demux1/2 -> 1_to_4_Bit_Demultiplexer(Bit_6)/3
  Demux1/1 -> 1_to_4_Bit_Demultiplexer(Bit_7)/3
  Byte_3/1 -> Bit to Integer Converter/1
  Byte_2/1 -> Bit to Integer Converter1/1
  Byte_1/1 -> Bit to Integer Converter2/1
  Byte_0/1 -> Bit to Integer Converter3/1
  1_to_4_Bit_Demultiplexer(Bit_0)/4 -> Byte_0/8
  1_to_4_Bit_Demultiplexer(Bit_0)/3 -> Byte_1/8
  1_to_4_Bit_Demultiplexer(Bit_0)/2 -> Byte_2/8
  1_to_4_Bit_Demultiplexer(Bit_0)/1 -> Byte_3/8
  1_to_4_Bit_Demultiplexer(Bit_1)/4 -> Byte_0/7
  1_to_4_Bit_Demultiplexer(Bit_1)/3 -> Byte_1/7
  1_to_4_Bit_Demultiplexer(Bit_1)/2 -> Byte_2/7
  1_to_4_Bit_Demultiplexer(Bit_1)/1 -> Byte_3/7
  1_to_4_Bit_Demultiplexer(Bit_2)/4 -> Byte_0/6
  1_to_4_Bit_Demultiplexer(Bit_2)/3 -> Byte_1/6
  1_to_4_Bit_Demultiplexer(Bit_2)/2 -> Byte_2/6
  1_to_4_Bit_Demultiplexer(Bit_2)/1 -> Byte_3/6
  1_to_4_Bit_Demultiplexer(Bit_3)/4 -> Byte_0/5
  1_to_4_Bit_Demultiplexer(Bit_3)/3 -> Byte_1/5
  1_to_4_Bit_Demultiplexer(Bit_3)/2 -> Byte_2/5
  1_to_4_Bit_Demultiplexer(Bit_3)/1 -> Byte_3/5
  1_to_4_Bit_Demultiplexer(Bit_4)/4 -> Byte_0/4
  1_to_4_Bit_Demultiplexer(Bit_4)/3 -> Byte_1/4
  1_to_4_Bit_Demultiplexer(Bit_4)/2 -> Byte_2/4
  1_to_4_Bit_Demultiplexer(Bit_4)/1 -> Byte_3/4
  1_to_4_Bit_Demultiplexer(Bit_5)/4 -> Byte_0/3
  1_to_4_Bit_Demultiplexer(Bit_5)/3 -> Byte_1/3
  1_to_4_Bit_Demultiplexer(Bit_5)/2 -> Byte_2/3
  1_to_4_Bit_Demultiplexer(Bit_5)/1 -> Byte_3/3
  1_to_4_Bit_Demultiplexer(Bit_6)/4 -> Byte_0/2
  1_to_4_Bit_Demultiplexer(Bit_6)/3 -> Byte_1/2
  1_to_4_Bit_Demultiplexer(Bit_6)/2 -> Byte_2/2
  1_to_4_Bit_Demultiplexer(Bit_6)/1 -> Byte_3/2
  1_to_4_Bit_Demultiplexer(Bit_7)/4 -> Byte_0/1
  1_to_4_Bit_Demultiplexer(Bit_7)/3 -> Byte_1/1
  1_to_4_Bit_Demultiplexer(Bit_7)/2 -> Byte_2/1
  1_to_4_Bit_Demultiplexer(Bit_7)/1 -> Byte_3/1
  Integer to Bit Converter7/1 -> Demux1/1
  Data_In(1B)/1 -> Integer to Bit Converter7/1
  Address_0(1b)/1 -> 1_to_4_Bit_Demultiplexer(Bit_7)/2, 1_to_4_Bit_Demultiplexer(Bit_3)/2, 1_to_4_Bit_Demultiplexer(Bit_2)/2, 1_to_4_Bit_Demultiplexer(Bit_1)/2, 1_to_4_Bit_Demultiplexer(Bit_0)/2, 1_to_4_Bit_Demultiplexer(Bit_4)/2, 1_to_4_Bit_Demultiplexer(Bit_5)/2, 1_to_4_Bit_Demultiplexer(Bit_6)/2
  Address_1(1b)/1 -> 1_to_4_Bit_Demultiplexer(Bit_7)/1, 1_to_4_Bit_Demultiplexer(Bit_0)/1, 1_to_4_Bit_Demultiplexer(Bit_1)/1, 1_to_4_Bit_Demultiplexer(Bit_2)/1, 1_to_4_Bit_Demultiplexer(Bit_3)/1, 1_to_4_Bit_Demultiplexer(Bit_4)/1, 1_to_4_Bit_Demultiplexer(Bit_5)/1, 1_to_4_Bit_Demultiplexer(Bit_6)/1
  Bit to Integer Converter1/1 -> Data_Out_2(1B)/1
  Bit to Integer Converter2/1 -> Data_Out_1(1B)/1
  Bit to Integer Converter3/1 -> Data_Out_0(1B)/1

== system Common_Library/Demultiplexers/1_to_8_Bit_Demultiplexer ==
  Address_2(1b) : Inport
  Address_1(1b) : Inport  Port=2
  Address_0(1b) : Inport  Port=3
  Data_In(1b) : Inport  Port=4
  Logical Operator{,1..7} (8 alike) : Logic  Inputs=4  IconShape=distinctive  AllPortsSameDT=off  OutDataTypeStr=boolean
  Logical Operator20 : Logic  Operator=NOT  Inputs=4  IconShape=distinctive  AllPortsSameDT=off  OutDataTypeStr=boolean
  Logical Operator21 : Logic  Operator=NOT  Inputs=4  IconShape=distinctive  AllPortsSameDT=off  OutDataTypeStr=boolean
  Logical Operator22 : Logic  Operator=NOT  Inputs=4  IconShape=distinctive  AllPortsSameDT=off  OutDataTypeStr=boolean
  Data_Out_7(1b) : Outport
  Data_Out_6(1b) : Outport  Port=2
  Data_Out_5(1b) : Outport  Port=3
  Data_Out_4(1b) : Outport  Port=4
  Data_Out_3(1b) : Outport  Port=5
  Data_Out_2(1b) : Outport  Port=6
  Data_Out_1(1b) : Outport  Port=7
  Data_Out_0(1b) : Outport  Port=8
  wires:
  Logical Operator6/1 -> Data_Out_1(1b)/1
  Logical Operator5/1 -> Data_Out_2(1b)/1
  Logical Operator4/1 -> Data_Out_3(1b)/1
  Logical Operator3/1 -> Data_Out_4(1b)/1
  Logical Operator2/1 -> Data_Out_5(1b)/1
  Logical Operator1/1 -> Data_Out_6(1b)/1
  Logical Operator/1 -> Data_Out_7(1b)/1
  Logical Operator22/1 -> Logical Operator1/4, Logical Operator3/4, Logical Operator5/4, Logical Operator7/4
  Address_0(1b)/1 -> Logical Operator2/4, Logical Operator4/4, Logical Operator6/4, Logical Operator/4, Logical Operator22/1
  Logical Operator21/1 -> Logical Operator2/3, Logical Operator3/3, Logical Operator6/3, Logical Operator7/3
  Address_1(1b)/1 -> Logical Operator1/3, Logical Operator4/3, Logical Operator5/3, Logical Operator/3, Logical Operator21/1
  Logical Operator20/1 -> Logical Operator4/2, Logical Operator5/2, Logical Operator6/2, Logical Operator7/2
  Address_2(1b)/1 -> Logical Operator1/2, Logical Operator2/2, Logical Operator3/2, Logical Operator/2, Logical Operator20/1
  Data_In(1b)/1 -> Logical Operator/1, Logical Operator1/1, Logical Operator2/1, Logical Operator3/1, Logical Operator4/1, Logical Operator5/1, Logical Operator6/1, Logical Operator7/1
  Logical Operator7/1 -> Data_Out_0(1b)/1

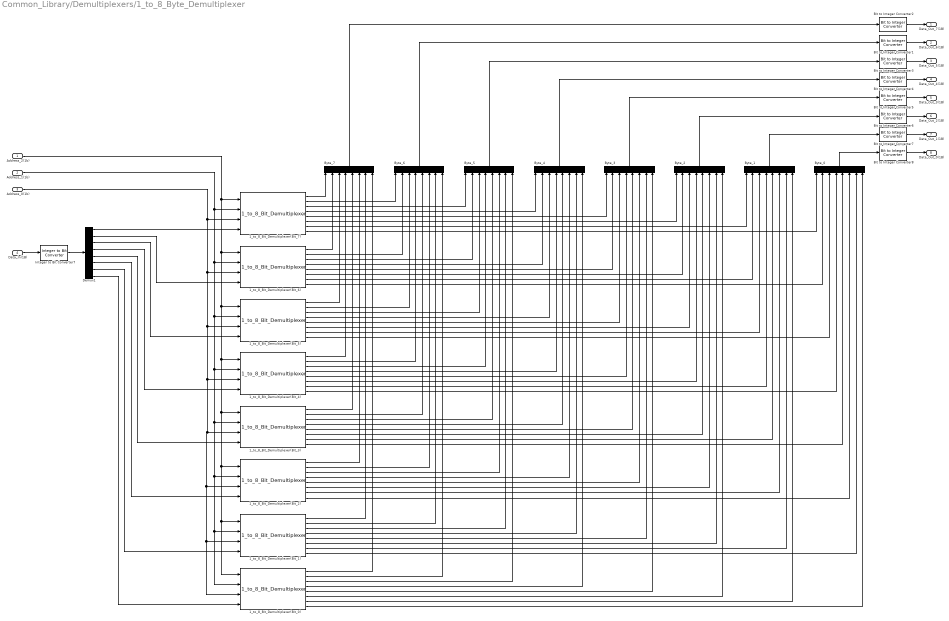
== system Common_Library/Demultiplexers/1_to_8_Byte_Demultiplexer ==
  Address_2(1b) : Inport
  Address_1(1b) : Inport  Port=2
  Address_0(1b) : Inport  Port=3
  Data_In(1B) : Inport  Port=4
  1_to_8_Bit_Demultiplexer(Bit_0) : Common_Library/Demultiplexers/1_to_8_Bit_Demultiplexer
  1_to_8_Bit_Demultiplexer(Bit_1) : Common_Library/Demultiplexers/1_to_8_Bit_Demultiplexer
  1_to_8_Bit_Demultiplexer(Bit_2) : Common_Library/Demultiplexers/1_to_8_Bit_Demultiplexer
  1_to_8_Bit_Demultiplexer(Bit_3) : Common_Library/Demultiplexers/1_to_8_Bit_Demultiplexer
  1_to_8_Bit_Demultiplexer(Bit_4) : Common_Library/Demultiplexers/1_to_8_Bit_Demultiplexer
  1_to_8_Bit_Demultiplexer(Bit_5) : Common_Library/Demultiplexers/1_to_8_Bit_Demultiplexer
  1_to_8_Bit_Demultiplexer(Bit_6) : Common_Library/Demultiplexers/1_to_8_Bit_Demultiplexer
  1_to_8_Bit_Demultiplexer(Bit_7) : Common_Library/Demultiplexers/1_to_8_Bit_Demultiplexer
  Bit to Integer Converter{1..8} (8 alike) : commutil2/Bit to Integer Converter  nbits=8  bitOrder=MSB first  signedOutputValues=Unsigned  outDtype=uint8  outDtypeSigned=Inherit via internal rule
  Byte_{0..7} (8 alike) : Mux  Inputs=8
  Demux1 : Demux  Outputs=8
  Integer to Bit Converter7 : commutil2/Integer to Bit Converter  nbits=8  signedInputValues=Unsigned  bitOrder=MSB first  outDtype=boolean
  Data_Out_7(1B) : Outport
  Data_Out_6(1B) : Outport  Port=2
  Data_Out_5(1B) : Outport  Port=3
  Data_Out_4(1B) : Outport  Port=4
  Data_Out_3(1B) : Outport  Port=5
  Data_Out_2(1B) : Outport  Port=6
  Data_Out_1(1B) : Outport  Port=7
  Data_Out_0(1B) : Outport  Port=8
  wires:
  Demux1/4 -> 1_to_8_Bit_Demultiplexer(Bit_4)/4
  Demux1/5 -> 1_to_8_Bit_Demultiplexer(Bit_3)/4
  Demux1/6 -> 1_to_8_Bit_Demultiplexer(Bit_2)/4
  Demux1/7 -> 1_to_8_Bit_Demultiplexer(Bit_1)/4
  Demux1/8 -> 1_to_8_Bit_Demultiplexer(Bit_0)/4
  Demux1/3 -> 1_to_8_Bit_Demultiplexer(Bit_5)/4
  Demux1/2 -> 1_to_8_Bit_Demultiplexer(Bit_6)/4
  Demux1/1 -> 1_to_8_Bit_Demultiplexer(Bit_7)/4
  Byte_7/1 -> Bit to Integer Converter2/1
  Byte_6/1 -> Bit to Integer Converter1/1
  Byte_5/1 -> Bit to Integer Converter3/1
  Byte_4/1 -> Bit to Integer Converter4/1
  Byte_3/1 -> Bit to Integer Converter5/1
  Byte_2/1 -> Bit to Integer Converter6/1
  Byte_1/1 -> Bit to Integer Converter7/1
  Byte_0/1 -> Bit to Integer Converter8/1
  1_to_8_Bit_Demultiplexer(Bit_0)/8 -> Byte_0/8
  1_to_8_Bit_Demultiplexer(Bit_0)/7 -> Byte_1/8
  1_to_8_Bit_Demultiplexer(Bit_0)/6 -> Byte_2/8
  1_to_8_Bit_Demultiplexer(Bit_0)/5 -> Byte_3/8
  1_to_8_Bit_Demultiplexer(Bit_0)/4 -> Byte_4/8
  1_to_8_Bit_Demultiplexer(Bit_0)/3 -> Byte_5/8
  1_to_8_Bit_Demultiplexer(Bit_0)/2 -> Byte_6/8
  1_to_8_Bit_Demultiplexer(Bit_0)/1 -> Byte_7/8
  1_to_8_Bit_Demultiplexer(Bit_1)/8 -> Byte_0/7
  1_to_8_Bit_Demultiplexer(Bit_1)/7 -> Byte_1/7
  1_to_8_Bit_Demultiplexer(Bit_1)/6 -> Byte_2/7
  1_to_8_Bit_Demultiplexer(Bit_1)/5 -> Byte_3/7
  1_to_8_Bit_Demultiplexer(Bit_1)/4 -> Byte_4/7
  1_to_8_Bit_Demultiplexer(Bit_1)/3 -> Byte_5/7
  1_to_8_Bit_Demultiplexer(Bit_1)/2 -> Byte_6/7
  1_to_8_Bit_Demultiplexer(Bit_1)/1 -> Byte_7/7
  1_to_8_Bit_Demultiplexer(Bit_2)/8 -> Byte_0/6
  1_to_8_Bit_Demultiplexer(Bit_2)/7 -> Byte_1/6
  1_to_8_Bit_Demultiplexer(Bit_2)/6 -> Byte_2/6
  1_to_8_Bit_Demultiplexer(Bit_2)/5 -> Byte_3/6
  1_to_8_Bit_Demultiplexer(Bit_2)/4 -> Byte_4/6
  1_to_8_Bit_Demultiplexer(Bit_2)/3 -> Byte_5/6
  1_to_8_Bit_Demultiplexer(Bit_2)/2 -> Byte_6/6
  1_to_8_Bit_Demultiplexer(Bit_2)/1 -> Byte_7/6
  1_to_8_Bit_Demultiplexer(Bit_3)/8 -> Byte_0/5
  1_to_8_Bit_Demultiplexer(Bit_3)/7 -> Byte_1/5
  1_to_8_Bit_Demultiplexer(Bit_3)/6 -> Byte_2/5
  1_to_8_Bit_Demultiplexer(Bit_3)/5 -> Byte_3/5
  1_to_8_Bit_Demultiplexer(Bit_3)/4 -> Byte_4/5
  1_to_8_Bit_Demultiplexer(Bit_3)/3 -> Byte_5/5
  1_to_8_Bit_Demultiplexer(Bit_3)/2 -> Byte_6/5
  1_to_8_Bit_Demultiplexer(Bit_3)/1 -> Byte_7/5
  1_to_8_Bit_Demultiplexer(Bit_4)/8 -> Byte_0/4
  1_to_8_Bit_Demultiplexer(Bit_4)/7 -> Byte_1/4
  1_to_8_Bit_Demultiplexer(Bit_4)/6 -> Byte_2/4
  1_to_8_Bit_Demultiplexer(Bit_4)/5 -> Byte_3/4
  1_to_8_Bit_Demultiplexer(Bit_4)/4 -> Byte_4/4
  1_to_8_Bit_Demultiplexer(Bit_4)/3 -> Byte_5/4
  1_to_8_Bit_Demultiplexer(Bit_4)/2 -> Byte_6/4
  1_to_8_Bit_Demultiplexer(Bit_4)/1 -> Byte_7/4
  1_to_8_Bit_Demultiplexer(Bit_5)/8 -> Byte_0/3
  1_to_8_Bit_Demultiplexer(Bit_5)/7 -> Byte_1/3
  1_to_8_Bit_Demultiplexer(Bit_5)/6 -> Byte_2/3
  1_to_8_Bit_Demultiplexer(Bit_5)/5 -> Byte_3/3
  1_to_8_Bit_Demultiplexer(Bit_5)/4 -> Byte_4/3
  1_to_8_Bit_Demultiplexer(Bit_5)/3 -> Byte_5/3
  1_to_8_Bit_Demultiplexer(Bit_5)/2 -> Byte_6/3
  1_to_8_Bit_Demultiplexer(Bit_5)/1 -> Byte_7/3
  1_to_8_Bit_Demultiplexer(Bit_6)/8 -> Byte_0/2
  1_to_8_Bit_Demultiplexer(Bit_6)/7 -> Byte_1/2
  1_to_8_Bit_Demultiplexer(Bit_6)/6 -> Byte_2/2
  1_to_8_Bit_Demultiplexer(Bit_6)/5 -> Byte_3/2
  1_to_8_Bit_Demultiplexer(Bit_6)/4 -> Byte_4/2
  1_to_8_Bit_Demultiplexer(Bit_6)/3 -> Byte_5/2
  1_to_8_Bit_Demultiplexer(Bit_6)/2 -> Byte_6/2
  1_to_8_Bit_Demultiplexer(Bit_6)/1 -> Byte_7/2
  1_to_8_Bit_Demultiplexer(Bit_7)/8 -> Byte_0/1
  1_to_8_Bit_Demultiplexer(Bit_7)/7 -> Byte_1/1
  1_to_8_Bit_Demultiplexer(Bit_7)/6 -> Byte_2/1
  1_to_8_Bit_Demultiplexer(Bit_7)/5 -> Byte_3/1
  1_to_8_Bit_Demultiplexer(Bit_7)/4 -> Byte_4/1
  1_to_8_Bit_Demultiplexer(Bit_7)/3 -> Byte_5/1
  1_to_8_Bit_Demultiplexer(Bit_7)/2 -> Byte_6/1
  1_to_8_Bit_Demultiplexer(Bit_7)/1 -> Byte_7/1
  Integer to Bit Converter7/1 -> Demux1/1
  Data_In(1B)/1 -> Integer to Bit Converter7/1
  Address_0(1b)/1 -> 1_to_8_Bit_Demultiplexer(Bit_7)/3, 1_to_8_Bit_Demultiplexer(Bit_6)/3, 1_to_8_Bit_Demultiplexer(Bit_5)/3, 1_to_8_Bit_Demultiplexer(Bit_0)/3, 1_to_8_Bit_Demultiplexer(Bit_1)/3, 1_to_8_Bit_Demultiplexer(Bit_2)/3, 1_to_8_Bit_Demultiplexer(Bit_3)/3, 1_to_8_Bit_Demultiplexer(Bit_4)/3
  Address_1(1b)/1 -> 1_to_8_Bit_Demultiplexer(Bit_7)/2, 1_to_8_Bit_Demultiplexer(Bit_0)/2, 1_to_8_Bit_Demultiplexer(Bit_1)/2, 1_to_8_Bit_Demultiplexer(Bit_2)/2, 1_to_8_Bit_Demultiplexer(Bit_3)/2, 1_to_8_Bit_Demultiplexer(Bit_4)/2, 1_to_8_Bit_Demultiplexer(Bit_5)/2, 1_to_8_Bit_Demultiplexer(Bit_6)/2
  Address_2(1b)/1 -> 1_to_8_Bit_Demultiplexer(Bit_7)/1, 1_to_8_Bit_Demultiplexer(Bit_0)/1, 1_to_8_Bit_Demultiplexer(Bit_1)/1, 1_to_8_Bit_Demultiplexer(Bit_2)/1, 1_to_8_Bit_Demultiplexer(Bit_3)/1, 1_to_8_Bit_Demultiplexer(Bit_4)/1, 1_to_8_Bit_Demultiplexer(Bit_5)/1, 1_to_8_Bit_Demultiplexer(Bit_6)/1
  Bit to Integer Converter8/1 -> Data_Out_0(1B)/1
  Bit to Integer Converter7/1 -> Data_Out_1(1B)/1
  Bit to Integer Converter6/1 -> Data_Out_2(1B)/1
  Bit to Integer Converter5/1 -> Data_Out_3(1B)/1
  Bit to Integer Converter4/1 -> Data_Out_4(1B)/1
  Bit to Integer Converter3/1 -> Data_Out_5(1B)/1
  Bit to Integer Converter1/1 -> Data_Out_6(1B)/1
  Bit to Integer Converter2/1 -> Data_Out_7(1B)/1
